simulink model "MdEnClear"  (R2024b)
settings: Solver=FixedStepDiscrete  StartTime=0.0  StopTime=10.0  FixedStep=0.01  RelTol=1e-3
undefined symbols (not defined in the file or in its folder): ClearBit, ModeState32_Clear
settings Model: ModifiedHistory=2024.7.11 V3.0.0 557模式流程V1.9  Creator=sn2xws  LastModifiedBy=sn55gm
settings SolverCC: AlgebraicLoopSolver=TrustRegion
settings DataIOCC: SaveFormat=StructureWithTime  ReturnWorkspaceOutputs=off
settings OptimizationCC: DefaultParameterBehavior=Inlined  EnhancedBackFolding=on  PassReuseOutputArgsAs=Individual arguments  ZeroExternalMemoryAtStartup=off  ZeroInternalMemoryAtStartup=off  OptimizeBlockOrder=speed  DifferentSizesBufferReuse=on  OptimizationCustomize=off  EfficientTunableParamExpr=on
settings DebuggingCC: ParameterTunabilityLossMsg=error  UnconnectedInputMsg=warning  UnconnectedOutputMsg=warning  UnconnectedLineMsg=warning  ArithmeticOperatorsInVariantConditions=warning
settings ModelReferenceCC: EnableRefExpFcnMdlSchedulingChecks=on  ModelReferenceNumInstancesAllowed=Single
settings SFSimCC: MATLABDynamicMemAlloc=off  CustomCodeUndefinedFunction=UseInterfaceOnly
settings RTWCC: Description=AUTOSAR  SystemTargetFile=autosar.tlc  GenCodeOnly=on  TemplateMakefile=ert_default_tmf  GenerateReport=on  IncludeHyperlinkInReport=on  LaunchReport=on  DataTypeReplacement=CDataTypesFixedWidth  GenerateTraceInfo=on  GenerateTraceReport=on  GenerateTraceReportSl=on  GenerateTraceReportSf=on  GenerateTraceReportEml=on  GenerateCodeMetricsReport=on  GPUComputeCapability=3.5
settings CodeAppCC: ForceParamTrailComments=on  IgnoreCustomStorageClasses=off  OperatorAnnotations=on  SimulinkDataObjDesc=on  SFDataObjDesc=on  InsertBlockDesc=on
settings STFCustomTargetCC: TargetLangStandard=C99 (ISO)  MultiwordLength=256  ParMdlRefBuildCompliant=on  CompOptLevelCompliant=on  IncludeMdlTerminateFcn=off  CombineOutputUpdateFcns=on  SuppressErrorStatus=on  ERTCustomFileBanners=on  SupportNonFinite=off  SupportComplex=off  SupportContinuousTime=off  SupportNonInlinedSFcns=off  RemoveResetFunc=on  MATLABClassNameForMDSCustomization=Simulink.SoftwareTarget.ERTCustomization  AutosarCompliant=on  UseToolchainInfoCompliant=on  LookupTableObjectStructAxisOrder=2,1,3,4,...  LUTObjectStructOrderEvenSpacing=Size,Table,Breakpoints  SystemTargetFile=autosar.tlc
settings ERTTargetCC: TargetLangStandard=C99 (ISO)  ConcurrentExecutionCompliant=off  IncludeMdlTerminateFcn=off  SuppressErrorStatus=on  SupportNonFinite=off  SupportComplex=off  ModelStepFunctionPrototypeControlCompliant=off  CPPClassGenCompliant=off  AutosarCompliant=on  LookupTableObjectStructAxisOrder=2,1,3,4,...  LUTObjectStructOrderEvenSpacing=Size,Table,Breakpoints  ERTCustomFileTemplate=example_file_process.tlc  ERTFilePackagingFormat=Compact  BooleanTrueId=TRUE  BooleanFalseId=FALSE  DynamicArrayContainerType=coder::array

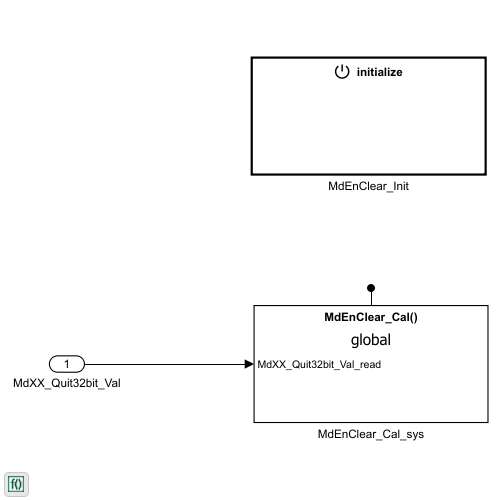
[thumbnail: Simulink's stored preview of the top-level diagram]
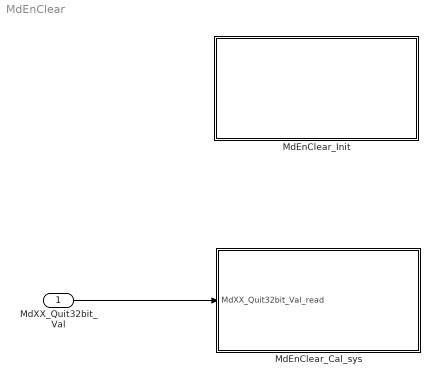
== system MdEnClear ==
  MdXX_Quit32bit_Val : Inport  OutDataTypeStr=uint32  PortDimensions=1
  MdEnClear_Cal_sys : Subsystem
  MdEnClear_Init : Subsystem
  wires:
  MdXX_Quit32bit_Val/1 -> MdEnClear_Cal_sys/1(MdXX_Quit32bit_Val_read)

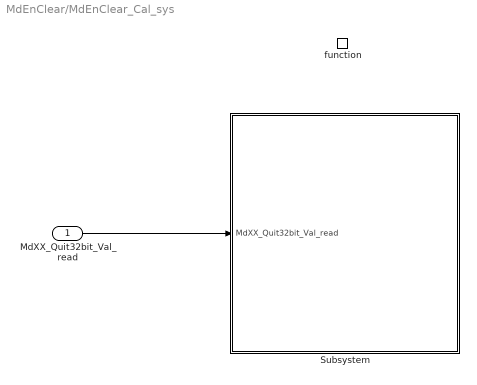
== system MdEnClear/MdEnClear_Cal_sys ==
  MdXX_Quit32bit_Val_read : Inport
  function : TriggerPort  TriggerType=function-call  IsSimulinkFunction=on  FunctionName=MdEnClear_Cal  VariantControl=(inherit)
  Subsystem : Subsystem
  wires:
  MdXX_Quit32bit_Val_read/1 -> Subsystem/1(MdXX_Quit32bit_Val_read)

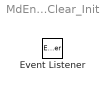
== system MdEnClear/MdEnClear_Init ==
  Event Listener : EventListener  EventName=reset

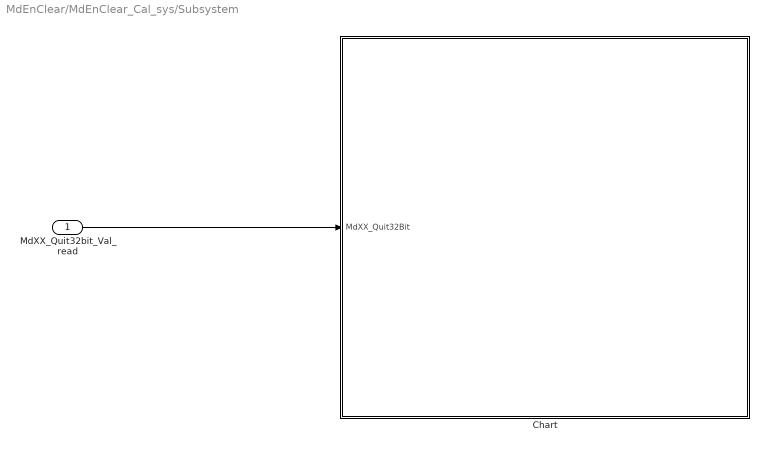
== system MdEnClear/MdEnClear_Cal_sys/Subsystem ==
  MdXX_Quit32bit_Val_read : Inport
  Chart : Stateflow chart  TreatAsAtomicUnit=on
  wires:
  MdXX_Quit32bit_Val_read/1 -> Chart/1(MdXX_Quit32Bit)

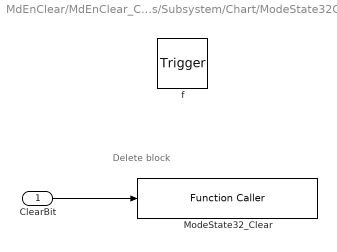
== system MdEnClear/MdEnClear_Cal_sys/Subsystem/Chart/ModeState32Clear ==
  note: Delete block
  ClearBit : Inport
  f : TriggerPort  TriggerType=function-call  VariantControl=(inherit)
      settings: CopyFcn=Stateflow.SLINSF.SimulinkMan.removeBlockPreDeleteFcn  PreDeleteFcn=Stateflow.SLINSF.SimulinkMan.unsafePredeleteFcn
  ModeState32_Clear : FunctionCaller  FunctionPrototype=ModeState32_Clear(ClearBit)  InputArgumentSpecifications=uint32(1)  OutputArgumentSpecifications=<Enter example>
  wires:
  ClearBit/1 -> ModeState32_Clear/1

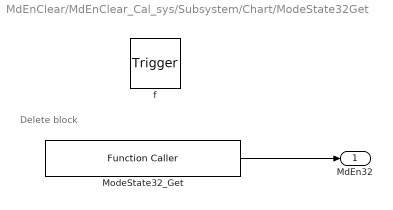
== system MdEnClear/MdEnClear_Cal_sys/Subsystem/Chart/ModeState32Get ==
  note: Delete block
  f : TriggerPort  TriggerType=function-call  VariantControl=(inherit)
      settings: CopyFcn=Stateflow.SLINSF.SimulinkMan.removeBlockPreDeleteFcn  PreDeleteFcn=Stateflow.SLINSF.SimulinkMan.unsafePredeleteFcn
  ModeState32_Get : FunctionCaller  FunctionPrototype=MdEn32 = ModeState32_Get()  InputArgumentSpecifications=<Enter example>  OutputArgumentSpecifications=uint32(1)
  MdEn32 : Outport  VectorParamsAs1DForOutWhenUnconnected=off
  wires:
  ModeState32_Get/1 -> MdEn32/1

== stateflow chart MdEnClear/MdEnClear_Cal_sys/Subsystem/Chart ==
  state ModeState32Clear(ClearBit) [function]
  state MdEn32 =ModeState32Get [function]
  (default) -> (junction 4)
  (junction 4) -> (junction 8) : {
      | MdXXEn32Bit = ModeState32Get();
      | ClearBit =(MdXX_Quit32Bit);
      | }
  (junction 8) -> (junction 19)
  (junction 19) -> (junction 21) [order 1] : [((MdXXEn32Bit&VIPAllBit)&&(MdXX_Quit32Bit&VIPAllBit))]
  (junction 19) -> (junction 25) [order 2]
  (junction 21) -> (junction 23) : {
      | ClearBit = ClearBit|(VIPLBit)|(VIPRBit);
      | }
  (junction 23) -> (junction 25)
  (junction 25) -> (junction 38)
  (junction 38) -> (junction 39) [order 1] : [((MdXXEn32Bit&LugAllBit)&&(MdXX_Quit32Bit&LugAllBit))]
  (junction 38) -> (junction 43) [order 2]
  (junction 39) -> (junction 41) : {
      | ClearBit = ClearBit |(LugLBit)|(LugRBit);
      | }
  (junction 41) -> (junction 43)
  (junction 43) -> (junction 97)
  (junction 97) -> (junction 99) [order 1] : [((MdXXEn32Bit&VIPExitAllBit)&&(MdXX_Quit32Bit&VIPExitAllBit))]
  (junction 97) -> (junction 103) [order 2]
  (junction 99) -> (junction 101) : {
      | ClearBit = ClearBit |(VIPLExitAllBit)|(VIPRExitAllBit);
      | }
  (junction 101) -> (junction 103)
  (junction 103) -> (junction 115)
  (junction 115) -> (junction 131) [order 1] : [((MdXXEn32Bit&32768)&&(MdXX_Quit32Bit&32768))]
  (junction 115) -> (junction 117) [order 2]
  (junction 131) -> (junction 130) : {
      | ClearBit = ClearBit |(8192)|(16384);
      | }
  (junction 130) -> (junction 117)
  (junction 117) -> (junction 63) : {
      | MdXXEn32Bit = MdXXEn32Bit&(~ClearBit);
      | }
  (junction 63) -> (junction 64) [order 1] : [(MdXXEn32Bit&VIPLBit)==0&&(MdXXEn32Bit&VIPRBit)==0]
  (junction 63) -> (junction 65) [order 2]
  (junction 64) -> (junction 66) : {
      | ClearBit =ClearBit|(VIPAllBit);
      | }
  (junction 66) -> (junction 65)
  (junction 65) -> (junction 74)
  (junction 74) -> (junction 76) [order 1] : [(MdXXEn32Bit&LugLBit)==0&&(MdXXEn32Bit&LugRBit)==0]
  (junction 74) -> (junction 75) [order 2]
  (junction 76) -> (junction 77) : {
      | ClearBit =ClearBit|(LugAllBit);
      | }
  (junction 77) -> (junction 75)
  (junction 75) -> (junction 106)
  (junction 106) -> (junction 108) [order 1] : [(MdXXEn32Bit&VIPLExitAllBit)==0&&(MdXXEn32Bit&VIPRExitAllBit)==0]
  (junction 106) -> (junction 112) [order 2]
  (junction 108) -> (junction 110) : {
      | ClearBit =ClearBit|(VIPExitAllBit);
      | }
  (junction 110) -> (junction 112)
  (junction 112) -> (junction 138)
  (junction 138) -> (junction 133) [order 1] : [(MdXXEn32Bit&8192)==0&&(MdXXEn32Bit&16384)==0]
  (junction 138) -> (junction 141) [order 2]
  (junction 133) -> (junction 135) : {
      | ClearBit =ClearBit|(32768);
      | }
  (junction 135) -> (junction 141)
  (junction 141) -> (junction 85) : {
      | ModeState32Clear(ClearBit);
      | }
  data: ClearBit function_input; MdEn32 function_output; MdXX_Quit32Bit input uint32; VIPLBit constant uint32 =512; VIPRBit constant uint32 =2048; LugLBit constant uint32 =128; LugRBit constant uint32 =256; LugAllBit constant uint32 =4; VIPAllBit constant uint32 =2; MdXXEn32Bit local uint32; ClearBit local uint32; VIPExitAllBit constant uint32 =268435456; VIPLExitAllBit constant uint32 =67108864; VIPRExitAllBit constant uint32 =134217728
